simulink model "BMS_SOC"  (R2025b)
settings: Solver=ode4  StartTime=0.0  StopTime=7000  FixedStep=0.1  MaxStep=1  RelTol=1e-3
undefined symbols (not defined in the file or in its folder): batt, cell, metadata
settings Model: SimulationMode=accelerator  Creator=39327  LastModifiedBy=faxio
settings DebuggingCC: UnconnectedInputMsg=warning  UnconnectedOutputMsg=warning  UnconnectedLineMsg=warning
settings ModelReferenceCC: EnableRefExpFcnMdlSchedulingChecks=on
settings RTWCC: GPUComputeCapability=3.5  DLArmComputeVersion=19.05

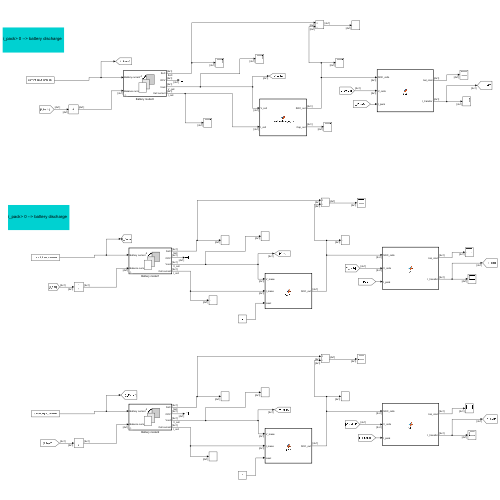
[thumbnail: Simulink's stored preview of the top-level diagram]
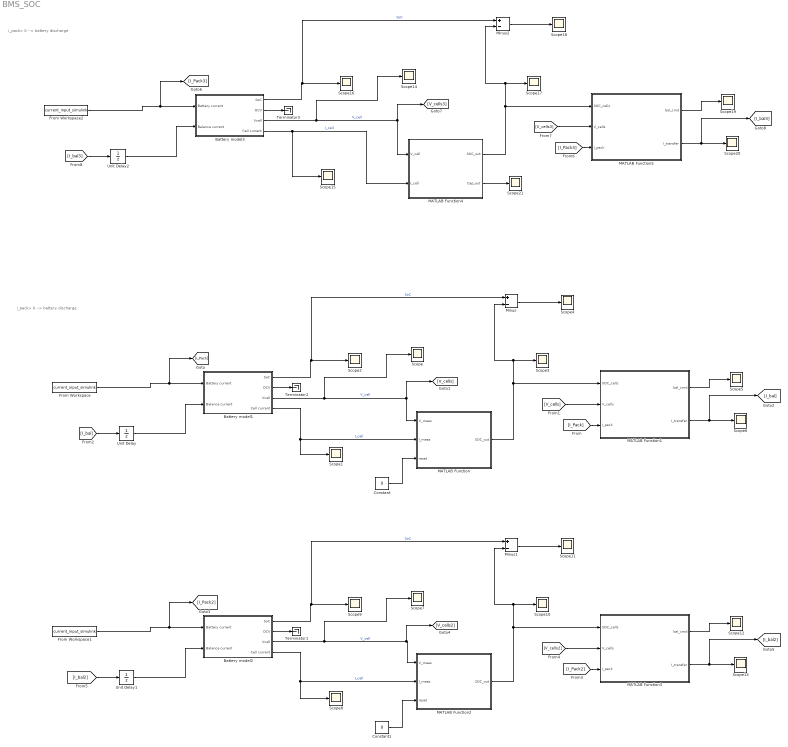
== system BMS_SOC ==
  note: i_pack> 0 --> battery discharge
  note: i_pack> 0 --> battery discharge
  Battery model1 : Subsystem  mask{Soc_init=batt.soc0, Qcell=batt.c_cell, R0_data=batt.r0, R1=batt.r1, C1=batt.c1, ocv_data=cell.ocv, soc_data=cell.soc}
      mask prompts: Soc_init "initial SoC [N_cell*1]"; Qcell "cell capacity [N_cell*1]"; R0_data "R0 [Ncell*soc_pnt]"; R1 "R1[not used here]"; C1 "C1[not used here]"; ocv_data "ocv_data [1*soc_pnt]"; soc_data "soc_data [1*soc_pnt]"
      mask DialogControl DescGroupVar Prompt: Battery model composed of Ncell
      mask DialogControl DescTextVar Prompt: the SoC varies in range 0-1.  Cell number is defined with the dimension of "cell capacity"[N_cell]
  Battery model2 : Subsystem  mask{Soc_init=batt.soc0, Qcell=batt.c_cell, R0_data=batt.r0, R1=batt.r1, C1=batt.c1, ocv_data=cell.ocv, soc_data=cell.soc}
      mask prompts: Soc_init "initial SoC [N_cell*1]"; Qcell "cell capacity [N_cell*1]"; R0_data "R0 [Ncell*soc_pnt]"; R1 "R1[not used here]"; C1 "C1[not used here]"; ocv_data "ocv_data [1*soc_pnt]"; soc_data "soc_data [1*soc_pnt]"
      mask DialogControl DescGroupVar Prompt: Battery model composed of Ncell
      mask DialogControl DescTextVar Prompt: the SoC varies in range 0-1.  Cell number is defined with the dimension of "cell capacity"[N_cell]
  Battery model3 : Subsystem  mask{Soc_init=batt.soc0, Qcell=batt.c_cell, R0_data=batt.r0, R1=batt.r1, C1=batt.c1, ocv_data=cell.ocv, soc_data=cell.soc}
      mask prompts: Soc_init "initial SoC [N_cell*1]"; Qcell "cell capacity [N_cell*1]"; R0_data "R0 [Ncell*soc_pnt]"; R1 "R1[not used here]"; C1 "C1[not used here]"; ocv_data "ocv_data [1*soc_pnt]"; soc_data "soc_data [1*soc_pnt]"
      mask DialogControl DescGroupVar Prompt: Battery model composed of Ncell
      mask DialogControl DescTextVar Prompt: the SoC varies in range 0-1.  Cell number is defined with the dimension of "cell capacity"[N_cell]
  Constant : Constant  Value=0
  Constant1 : Constant  Value=0
  From Workspace : FromWorkspace  VariableName=current_input_simulink  SampleTime=1
  From Workspace1 : FromWorkspace  VariableName=current_input_simulink  SampleTime=1
  From Workspace2 : FromWorkspace  VariableName=current_input_simulink  SampleTime=1
  MATLAB Function : MATLAB Function  TreatAsAtomicUnit=on
  MATLAB Function1 : MATLAB Function  TreatAsAtomicUnit=on  SystemSampleTime=0.1
  MATLAB Function2 : MATLAB Function  TreatAsAtomicUnit=on
  MATLAB Function3 : MATLAB Function  TreatAsAtomicUnit=on  SystemSampleTime=0.1
  MATLAB Function4 : MATLAB Function  TreatAsAtomicUnit=on
  MATLAB Function5 : MATLAB Function  TreatAsAtomicUnit=on  SystemSampleTime=0.1
  Minus : Sum  Inputs=+-
  Minus1 : Sum  Inputs=+-
  Minus2 : Sum  Inputs=+-
  Scope{,1..21} (22 alike) : Scope
      Scope settings: ActiveDisplayYMinimum=3.2688273744129139  ActiveDisplayYMaximum=4.3528683057854645
      Scope1 settings: ActiveDisplayYMinimum=-4.7084210256264356  ActiveDisplayYMaximum=4.9676023361807147
      Scope10 settings: ActiveDisplayYMinimum=-0.1  ActiveDisplayYMaximum=1.1  DataLoggingVariableName=ScopeData7
      Scope11 settings: ActiveDisplayYMinimum=-0.15496450956014618  ActiveDisplayYMaximum=0.21781817172296922  DataLoggingVariableName=ScopeData8
      Scope12 settings: ActiveDisplayYMinimum=-1.2378278494765407  ActiveDisplayYMaximum=1.1192335784275058  DataLoggingVariableName=ScopeData9
      Scope13 settings: ActiveDisplayYMinimum=-1.1600000000000001  ActiveDisplayYMaximum=1.24  DataLoggingVariableName=ScopeData10
      Scope14 settings: ActiveDisplayYMinimum=3.2688273744129139  ActiveDisplayYMaximum=4.3528683057854645  DataLoggingVariableName=ScopeData14
      Scope15 settings: ActiveDisplayYMinimum=-4.7084210256264356  ActiveDisplayYMaximum=4.9676023361807147  DataLoggingVariableName=ScopeData15
      Scope16 settings: ActiveDisplayYMinimum=-0.1  ActiveDisplayYMaximum=1.1  DataLoggingVariableName=ScopeData16
      Scope17 settings: ActiveDisplayYMinimum=0.92795123772963251  ActiveDisplayYMaximum=1.0349099222905718  DataLoggingVariableName=ScopeData17
      Scope18 settings: ActiveDisplayYMinimum=-0.30283794359420108  ActiveDisplayYMaximum=0.25636016397696909  DataLoggingVariableName=ScopeData18
      Scope19 settings: ActiveDisplayYMinimum=-1.2378278494765407  ActiveDisplayYMaximum=1.1192335784275058  DataLoggingVariableName=ScopeData19
      Scope2 settings: ActiveDisplayYMinimum=-0.1  ActiveDisplayYMaximum=1.1  DataLoggingVariableName=ScopeData2
      Scope20 settings: ActiveDisplayYMinimum=-0.32080851306321917  ActiveDisplayYMaximum=0.28672639786307896  DataLoggingVariableName=ScopeData20
      Scope21 settings: ActiveDisplayYMinimum=-2.039376682993602E+9  ActiveDisplayYMaximum=1.6277220397698671E+10  DataLoggingVariableName=ScopeData21
      Scope3 settings: ActiveDisplayYMinimum=-0.1  ActiveDisplayYMaximum=1.1  DataLoggingVariableName=ScopeData3
      Scope4 settings: ActiveDisplayYMinimum=-0.015721734219682579  ActiveDisplayYMaximum=0.063471743751515083  DataLoggingVariableName=ScopeData4
      Scope5 settings: ActiveDisplayYMinimum=-1.2378278494765407  ActiveDisplayYMaximum=1.1192335784275058  DataLoggingVariableName=ScopeData5
      Scope6 settings: ActiveDisplayYMinimum=-0.32080851306321917  ActiveDisplayYMaximum=0.28672639786307896  DataLoggingVariableName=ScopeData6
      Scope7 settings: ActiveDisplayYMinimum=3.2688273744129139  ActiveDisplayYMaximum=4.3528683057854645  DataLoggingVariableName=ScopeData11
      Scope8 settings: ActiveDisplayYMinimum=-4.7084210256264356  ActiveDisplayYMaximum=4.9676023361807147  DataLoggingVariableName=ScopeData12
      Scope9 settings: ActiveDisplayYMinimum=-0.1  ActiveDisplayYMaximum=1.1  DataLoggingVariableName=ScopeData13
  Terminator1 : Terminator
  Terminator2 : Terminator
  Terminator3 : Terminator
  Unit Delay : UnitDelay  SampleTime=-1  HasFrameUpgradeWarning=on
  Unit Delay1 : UnitDelay  SampleTime=-1  HasFrameUpgradeWarning=on
  Unit Delay2 : UnitDelay  SampleTime=-1  HasFrameUpgradeWarning=on
  wires:
  Battery model1/2(OCV) -> Terminator2/1
  From Workspace/1 -> [I_Pack], Battery model1/1(Battery current)
  Battery model1/1(SoC) -> Minus/1, Scope2/1  "SoC"
  [I_bal] -> Unit Delay/1
  Battery model1/3(Vcell) -> Scope/1, [V_cells], MATLAB Function/1(V_meas)  "V_cell"
  Battery model1/4(Cell current) -> Scope1/1, MATLAB Function/2(I_meas)  "I_cell"
  MATLAB Function/1(SOC_out) -> Minus/2, Scope3/1, MATLAB Function1/1(SOC_cells)
  [I_Pack] -> MATLAB Function1/3(I_pack)
  [V_cells] -> MATLAB Function1/2(V_cells)
  MATLAB Function1/2(I_transfer) -> Scope6/1, [I_bal]
  MATLAB Function1/1(bal_cmd) -> Scope5/1
  Unit Delay/1 -> Battery model1/2(Balance current)
  Minus/1 -> Scope4/1
  Minus1/1 -> Scope11/1
  [I_Pack2] -> MATLAB Function3/3(I_pack)
  [V_cells2] -> MATLAB Function3/2(V_cells)
  Battery model2/3(Vcell) -> Scope7/1, MATLAB Function2/1(V_meas), [V_cells2]  "V_cell"
  Battery model2/4(Cell current) -> MATLAB Function2/2(I_meas), Scope8/1  "I_cell"
  From Workspace1/1 -> [I_Pack2], Battery model2/1(Battery current)
  [I_bal2] -> Unit Delay1/1
  MATLAB Function3/1(bal_cmd) -> Scope12/1
  Unit Delay1/1 -> Battery model2/2(Balance current)
  MATLAB Function2/1(SOC_out) -> Minus1/2, Scope10/1, MATLAB Function3/1(SOC_cells)
  Battery model2/2(OCV) -> Terminator1/1
  Battery model2/1(SoC) -> Minus1/1, Scope9/1  "SoC"
  Constant1/1 -> MATLAB Function2/3(reset)
  MATLAB Function3/2(I_transfer) -> Scope13/1, [I_bal2]
  MATLAB Function5/2(I_transfer) -> Scope20/1, [I_bal3]
  Battery model3/3(Vcell) -> Scope14/1, [V_cells3], MATLAB Function4/1(V_cell)  "V_cell"
  [I_bal3] -> Unit Delay2/1
  Unit Delay2/1 -> Battery model3/2(Balance current)
  From Workspace2/1 -> [I_Pack3], Battery model3/1(Battery current)
  Battery model3/4(Cell current) -> MATLAB Function4/2(I_cell), Scope15/1  "I_cell"
  [V_cells3] -> MATLAB Function5/2(V_cells)
  [I_Pack3] -> MATLAB Function5/3(I_pack)
  MATLAB Function5/1(bal_cmd) -> Scope19/1
  MATLAB Function4/1(SOC_out) -> Minus2/2, Scope17/1, MATLAB Function5/1(SOC_cells)
  Battery model3/1(SoC) -> Minus2/1, Scope16/1  "SoC"
  Minus2/1 -> Scope18/1
  Battery model3/2(OCV) -> Terminator3/1
  Constant/1 -> MATLAB Function/3(reset)
  MATLAB Function4/2(Cap_out) -> Scope21/1

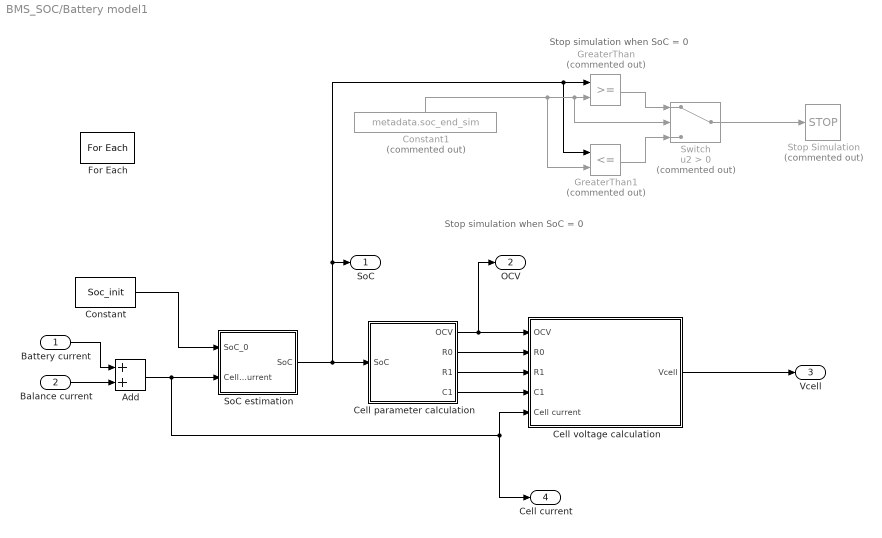
== system BMS_SOC/Battery model1 ==
  note: Stop simulation when SoC = 0
  note: Stop simulation when SoC = 0
  Battery current : Inport
  Balance current : Inport  Port=2  Partition=on  PartitionDimension=1  PartitionWidth=1  PartitionOffset=0
  Add : Sum
  Cell parameter calculation : Subsystem
  Cell voltage calculation : Subsystem
  Constant : Constant  Value=Soc_init
  Constant1 : Constant  Commented=on  Value=metadata.soc_end_sim
  For Each : ForEach  DisableCoverage=on  IterateSubsysMaskParameter=on,on,on,off,off,off,off
  GreaterThan : RelationalOperator  Commented=on  OutDataTypeStr=boolean  RndMeth=Simplest  InputSameDT=off
  GreaterThan1 : RelationalOperator  Commented=on  Operator=<=  OutDataTypeStr=boolean  RndMeth=Simplest  InputSameDT=off
  SoC estimation : Subsystem
  Stop Simulation : Stop  Commented=on
  Switch : Switch  Commented=on  Criteria=u2 > Threshold  SaturateOnIntegerOverflow=off  InputSameDT=off
  SoC : Outport  ConcatenationDimension=1
  OCV : Outport  Port=2  ConcatenationDimension=1
  Vcell : Outport  Port=3  ConcatenationDimension=1
  Cell current : Outport  Port=4  ConcatenationDimension=1
  wires:
  Add/1 -> Cell voltage calculation/5(Cell current), Cell current/1, SoC estimation/2(Cell current)
  Constant/1 -> SoC estimation/1(SoC_0)
  SoC estimation/1(SoC) -> GreaterThan/1, GreaterThan1/1, SoC/1, Cell parameter calculation/1(SoC)
  Cell parameter calculation/4(C1) -> Cell voltage calculation/4(C1)
  Cell parameter calculation/3(R1) -> Cell voltage calculation/3(R1)
  Cell parameter calculation/2(R0) -> Cell voltage calculation/2(R0)
  Cell parameter calculation/1(OCV) -> OCV/1, Cell voltage calculation/1(OCV)
  Cell voltage calculation/1(Vcell) -> Vcell/1
  Battery current/1 -> Add/1
  Balance current/1 -> Add/2
  Constant1/1 -> GreaterThan/2, Switch/2, GreaterThan1/2
  Switch/1 -> Stop Simulation/1
  GreaterThan/1 -> Switch/1
  GreaterThan1/1 -> Switch/3

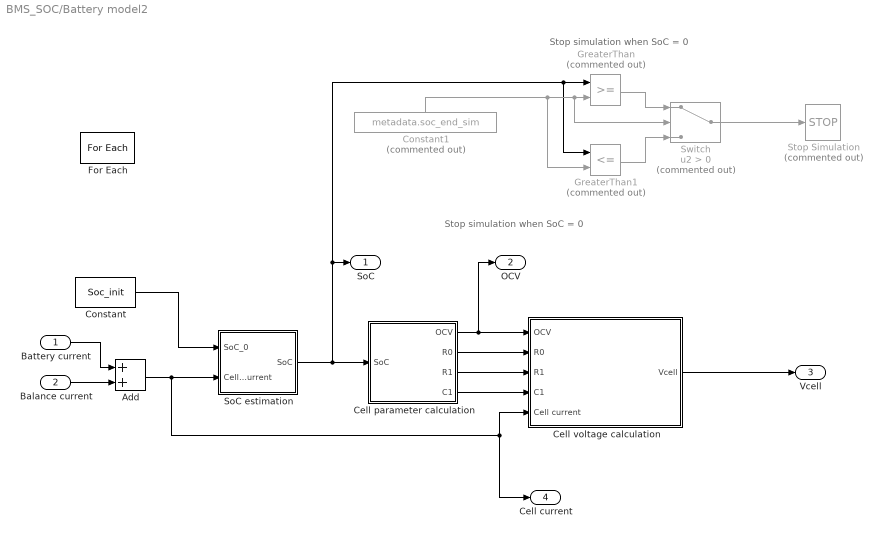
== system BMS_SOC/Battery model2 ==
  note: Stop simulation when SoC = 0
  note: Stop simulation when SoC = 0
  Battery current : Inport
  Balance current : Inport  Port=2  Partition=on  PartitionDimension=1  PartitionWidth=1  PartitionOffset=0
  Add : Sum
  Cell parameter calculation : Subsystem
  Cell voltage calculation : Subsystem
  Constant : Constant  Value=Soc_init
  Constant1 : Constant  Commented=on  Value=metadata.soc_end_sim
  For Each : ForEach  DisableCoverage=on  IterateSubsysMaskParameter=on,on,on,off,off,off,off
  GreaterThan : RelationalOperator  Commented=on  OutDataTypeStr=boolean  RndMeth=Simplest  InputSameDT=off
  GreaterThan1 : RelationalOperator  Commented=on  Operator=<=  OutDataTypeStr=boolean  RndMeth=Simplest  InputSameDT=off
  SoC estimation : Subsystem
  Stop Simulation : Stop  Commented=on
  Switch : Switch  Commented=on  Criteria=u2 > Threshold  SaturateOnIntegerOverflow=off  InputSameDT=off
  SoC : Outport  ConcatenationDimension=1
  OCV : Outport  Port=2  ConcatenationDimension=1
  Vcell : Outport  Port=3  ConcatenationDimension=1
  Cell current : Outport  Port=4  ConcatenationDimension=1
  wires:
  Add/1 -> Cell voltage calculation/5(Cell current), Cell current/1, SoC estimation/2(Cell current)
  Constant/1 -> SoC estimation/1(SoC_0)
  SoC estimation/1(SoC) -> GreaterThan/1, GreaterThan1/1, SoC/1, Cell parameter calculation/1(SoC)
  Cell parameter calculation/4(C1) -> Cell voltage calculation/4(C1)
  Cell parameter calculation/3(R1) -> Cell voltage calculation/3(R1)
  Cell parameter calculation/2(R0) -> Cell voltage calculation/2(R0)
  Cell parameter calculation/1(OCV) -> OCV/1, Cell voltage calculation/1(OCV)
  Cell voltage calculation/1(Vcell) -> Vcell/1
  Battery current/1 -> Add/1
  Balance current/1 -> Add/2
  Constant1/1 -> GreaterThan/2, Switch/2, GreaterThan1/2
  Switch/1 -> Stop Simulation/1
  GreaterThan/1 -> Switch/1
  GreaterThan1/1 -> Switch/3

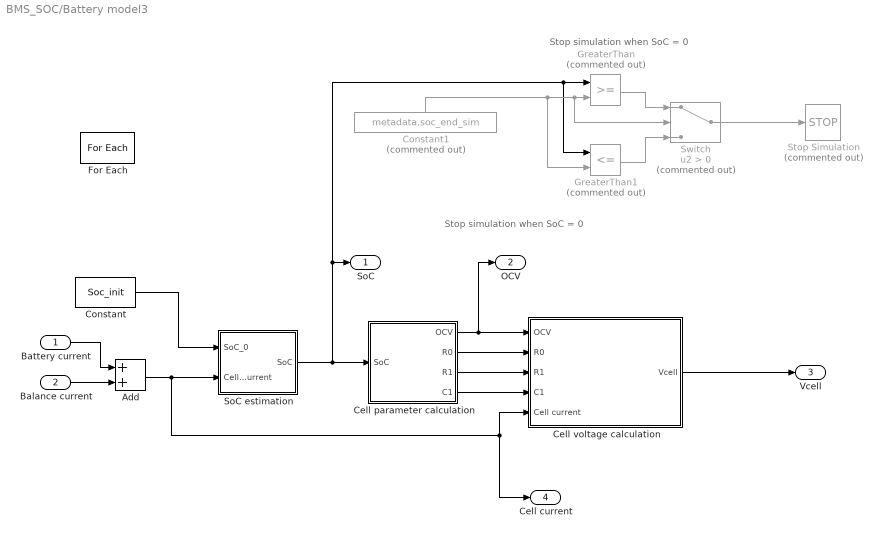
== system BMS_SOC/Battery model3 ==
  note: Stop simulation when SoC = 0
  note: Stop simulation when SoC = 0
  Battery current : Inport
  Balance current : Inport  Port=2  Partition=on  PartitionDimension=1  PartitionWidth=1  PartitionOffset=0
  Add : Sum
  Cell parameter calculation : Subsystem
  Cell voltage calculation : Subsystem
  Constant : Constant  Value=Soc_init
  Constant1 : Constant  Commented=on  Value=metadata.soc_end_sim
  For Each : ForEach  DisableCoverage=on  IterateSubsysMaskParameter=on,on,on,off,off,off,off
  GreaterThan : RelationalOperator  Commented=on  OutDataTypeStr=boolean  RndMeth=Simplest  InputSameDT=off
  GreaterThan1 : RelationalOperator  Commented=on  Operator=<=  OutDataTypeStr=boolean  RndMeth=Simplest  InputSameDT=off
  SoC estimation : Subsystem
  Stop Simulation : Stop  Commented=on
  Switch : Switch  Commented=on  Criteria=u2 > Threshold  SaturateOnIntegerOverflow=off  InputSameDT=off
  SoC : Outport  ConcatenationDimension=1
  OCV : Outport  Port=2  ConcatenationDimension=1
  Vcell : Outport  Port=3  ConcatenationDimension=1
  Cell current : Outport  Port=4  ConcatenationDimension=1
  wires:
  Add/1 -> Cell voltage calculation/5(Cell current), Cell current/1, SoC estimation/2(Cell current)
  Constant/1 -> SoC estimation/1(SoC_0)
  SoC estimation/1(SoC) -> GreaterThan/1, GreaterThan1/1, SoC/1, Cell parameter calculation/1(SoC)
  Cell parameter calculation/4(C1) -> Cell voltage calculation/4(C1)
  Cell parameter calculation/3(R1) -> Cell voltage calculation/3(R1)
  Cell parameter calculation/2(R0) -> Cell voltage calculation/2(R0)
  Cell parameter calculation/1(OCV) -> OCV/1, Cell voltage calculation/1(OCV)
  Cell voltage calculation/1(Vcell) -> Vcell/1
  Battery current/1 -> Add/1
  Balance current/1 -> Add/2
  Constant1/1 -> GreaterThan/2, Switch/2, GreaterThan1/2
  Switch/1 -> Stop Simulation/1
  GreaterThan/1 -> Switch/1
  GreaterThan1/1 -> Switch/3

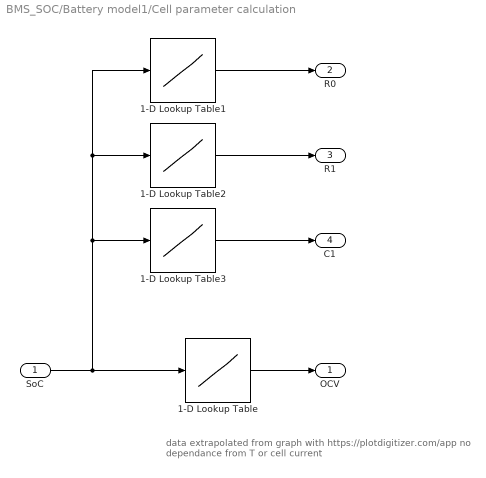
== system BMS_SOC/Battery model1/Cell parameter calculation ==
  note: data extrapolated from graph with https://plotdigitizer.com/app
      |
      | no dependance from T or cell current
  SoC : Inport
  1-D Lookup Table : Lookup_n-D  NumberOfTableDimensions=1  BreakpointsForDimension1=cell.soc  Table=cell.ocv  InternalRulePriority=Speed  RndMeth=Simplest
  1-D Lookup Table1 : Lookup_n-D  NumberOfTableDimensions=1  BreakpointsForDimension1=cell.soc  Table=cell.r0  InternalRulePriority=Speed  RndMeth=Simplest
  1-D Lookup Table2 : Lookup_n-D  NumberOfTableDimensions=1  BreakpointsForDimension1=cell.soc  Table=cell.r1  InternalRulePriority=Speed  RndMeth=Simplest
  1-D Lookup Table3 : Lookup_n-D  NumberOfTableDimensions=1  BreakpointsForDimension1=cell.soc  Table=cell.c1  InternalRulePriority=Speed  RndMeth=Simplest
  OCV : Outport
  R0 : Outport  Port=2
  R1 : Outport  Port=3
  C1 : Outport  Port=4
  wires:
  1-D Lookup Table/1 -> OCV/1
  SoC/1 -> 1-D Lookup Table3/1, 1-D Lookup Table2/1, 1-D Lookup Table1/1, 1-D Lookup Table/1
  1-D Lookup Table1/1 -> R0/1
  1-D Lookup Table3/1 -> C1/1
  1-D Lookup Table2/1 -> R1/1

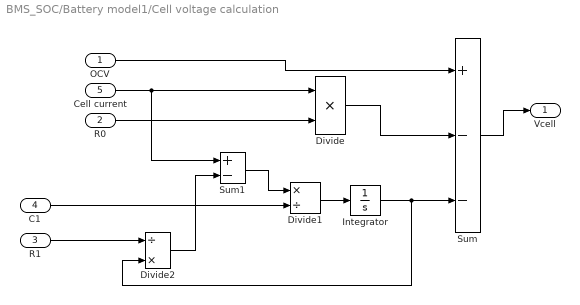
== system BMS_SOC/Battery model1/Cell voltage calculation ==
  OCV : Inport
  R0 : Inport  Port=2
  R1 : Inport  Port=3
  C1 : Inport  Port=4
  Cell current : Inport  Port=5
  Divide : Product  Inputs=**
  Divide1 : Product  Inputs=*/
  Divide2 : Product  Inputs=/*
  Integrator : Integrator
  Sum : Sum  Inputs=+--
  Sum1 : Sum  Inputs=+-
  Vcell : Outport
  wires:
  Sum/1 -> Vcell/1
  OCV/1 -> Sum/1
  Divide/1 -> Sum/2
  Cell current/1 -> Sum1/1, Divide/1
  R0/1 -> Divide/2
  Divide1/1 -> Integrator/1
  Integrator/1 -> Sum/3, Divide2/2
  Sum1/1 -> Divide1/1
  Divide2/1 -> Sum1/2
  C1/1 -> Divide1/2
  R1/1 -> Divide2/1

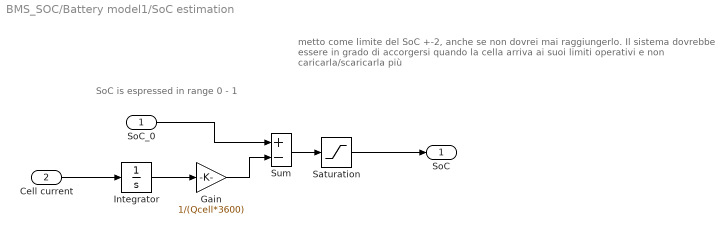
== system BMS_SOC/Battery model1/SoC estimation ==
  note: metto come limite del SoC +-2, anche se non dovrei mai raggiungerlo. Il sistema dovrebbe essere in grado di accorgersi quando la cella arriva ai suoi limiti operativi e non caricarla/scaricarla più
  note: SoC is espressed in range 0 - 1
  SoC_0 : Inport
  Cell current : Inport  Port=2
  Gain : Gain  Gain=1/(Qcell*3600)
  Integrator : Integrator
  Saturation : Saturate  UpperLimit=2  LowerLimit=-2
  Sum : Sum  Inputs=+-
  SoC : Outport
  wires:
  Saturation/1 -> SoC/1
  Integrator/1 -> Gain/1
  Cell current/1 -> Integrator/1
  Sum/1 -> Saturation/1
  Gain/1 -> Sum/2
  SoC_0/1 -> Sum/1

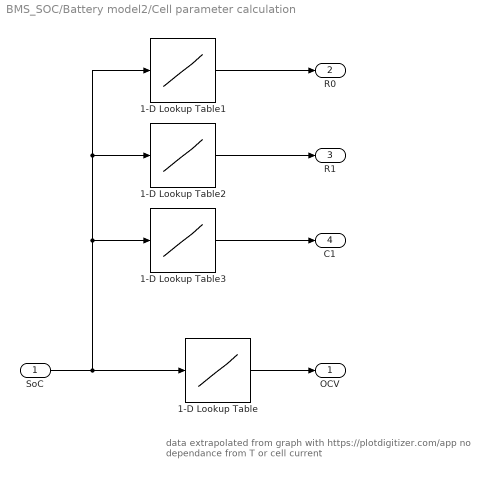
== system BMS_SOC/Battery model2/Cell parameter calculation ==
  note: data extrapolated from graph with https://plotdigitizer.com/app
      |
      | no dependance from T or cell current
  SoC : Inport
  1-D Lookup Table : Lookup_n-D  NumberOfTableDimensions=1  BreakpointsForDimension1=cell.soc  Table=cell.ocv  InternalRulePriority=Speed  RndMeth=Simplest
  1-D Lookup Table1 : Lookup_n-D  NumberOfTableDimensions=1  BreakpointsForDimension1=cell.soc  Table=cell.r0  InternalRulePriority=Speed  RndMeth=Simplest
  1-D Lookup Table2 : Lookup_n-D  NumberOfTableDimensions=1  BreakpointsForDimension1=cell.soc  Table=cell.r1  InternalRulePriority=Speed  RndMeth=Simplest
  1-D Lookup Table3 : Lookup_n-D  NumberOfTableDimensions=1  BreakpointsForDimension1=cell.soc  Table=cell.c1  InternalRulePriority=Speed  RndMeth=Simplest
  OCV : Outport
  R0 : Outport  Port=2
  R1 : Outport  Port=3
  C1 : Outport  Port=4
  wires:
  1-D Lookup Table/1 -> OCV/1
  SoC/1 -> 1-D Lookup Table3/1, 1-D Lookup Table2/1, 1-D Lookup Table1/1, 1-D Lookup Table/1
  1-D Lookup Table1/1 -> R0/1
  1-D Lookup Table3/1 -> C1/1
  1-D Lookup Table2/1 -> R1/1

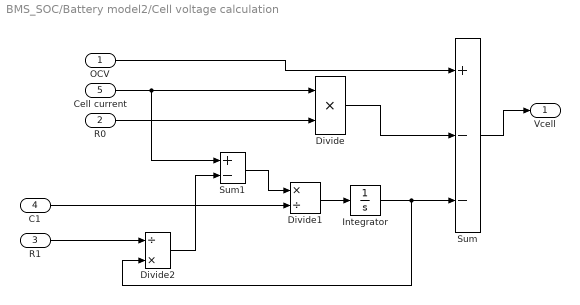
== system BMS_SOC/Battery model2/Cell voltage calculation ==
  OCV : Inport
  R0 : Inport  Port=2
  R1 : Inport  Port=3
  C1 : Inport  Port=4
  Cell current : Inport  Port=5
  Divide : Product  Inputs=**
  Divide1 : Product  Inputs=*/
  Divide2 : Product  Inputs=/*
  Integrator : Integrator
  Sum : Sum  Inputs=+--
  Sum1 : Sum  Inputs=+-
  Vcell : Outport
  wires:
  Sum/1 -> Vcell/1
  OCV/1 -> Sum/1
  Divide/1 -> Sum/2
  Cell current/1 -> Sum1/1, Divide/1
  R0/1 -> Divide/2
  Divide1/1 -> Integrator/1
  Integrator/1 -> Sum/3, Divide2/2
  Sum1/1 -> Divide1/1
  Divide2/1 -> Sum1/2
  C1/1 -> Divide1/2
  R1/1 -> Divide2/1

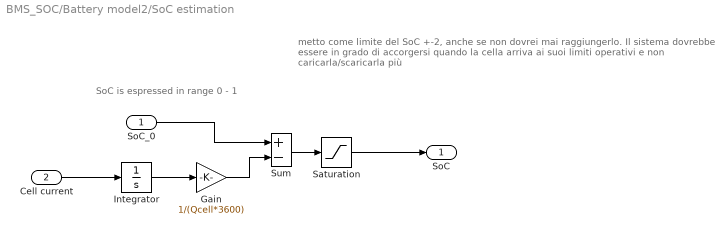
== system BMS_SOC/Battery model2/SoC estimation ==
  note: metto come limite del SoC +-2, anche se non dovrei mai raggiungerlo. Il sistema dovrebbe essere in grado di accorgersi quando la cella arriva ai suoi limiti operativi e non caricarla/scaricarla più
  note: SoC is espressed in range 0 - 1
  SoC_0 : Inport
  Cell current : Inport  Port=2
  Gain : Gain  Gain=1/(Qcell*3600)
  Integrator : Integrator
  Saturation : Saturate  UpperLimit=2  LowerLimit=-2
  Sum : Sum  Inputs=+-
  SoC : Outport
  wires:
  Saturation/1 -> SoC/1
  Integrator/1 -> Gain/1
  Cell current/1 -> Integrator/1
  Sum/1 -> Saturation/1
  Gain/1 -> Sum/2
  SoC_0/1 -> Sum/1

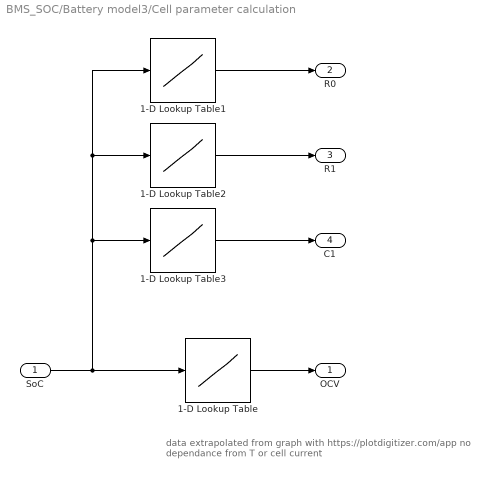
== system BMS_SOC/Battery model3/Cell parameter calculation ==
  note: data extrapolated from graph with https://plotdigitizer.com/app
      |
      | no dependance from T or cell current
  SoC : Inport
  1-D Lookup Table : Lookup_n-D  NumberOfTableDimensions=1  BreakpointsForDimension1=cell.soc  Table=cell.ocv  InternalRulePriority=Speed  RndMeth=Simplest
  1-D Lookup Table1 : Lookup_n-D  NumberOfTableDimensions=1  BreakpointsForDimension1=cell.soc  Table=cell.r0  InternalRulePriority=Speed  RndMeth=Simplest
  1-D Lookup Table2 : Lookup_n-D  NumberOfTableDimensions=1  BreakpointsForDimension1=cell.soc  Table=cell.r1  InternalRulePriority=Speed  RndMeth=Simplest
  1-D Lookup Table3 : Lookup_n-D  NumberOfTableDimensions=1  BreakpointsForDimension1=cell.soc  Table=cell.c1  InternalRulePriority=Speed  RndMeth=Simplest
  OCV : Outport
  R0 : Outport  Port=2
  R1 : Outport  Port=3
  C1 : Outport  Port=4
  wires:
  1-D Lookup Table/1 -> OCV/1
  SoC/1 -> 1-D Lookup Table3/1, 1-D Lookup Table2/1, 1-D Lookup Table1/1, 1-D Lookup Table/1
  1-D Lookup Table1/1 -> R0/1
  1-D Lookup Table3/1 -> C1/1
  1-D Lookup Table2/1 -> R1/1

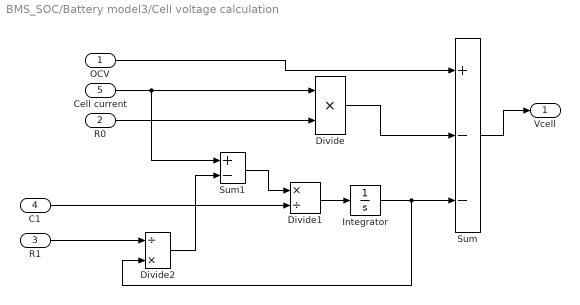
== system BMS_SOC/Battery model3/Cell voltage calculation ==
  OCV : Inport
  R0 : Inport  Port=2
  R1 : Inport  Port=3
  C1 : Inport  Port=4
  Cell current : Inport  Port=5
  Divide : Product  Inputs=**
  Divide1 : Product  Inputs=*/
  Divide2 : Product  Inputs=/*
  Integrator : Integrator
  Sum : Sum  Inputs=+--
  Sum1 : Sum  Inputs=+-
  Vcell : Outport
  wires:
  Sum/1 -> Vcell/1
  OCV/1 -> Sum/1
  Divide/1 -> Sum/2
  Cell current/1 -> Sum1/1, Divide/1
  R0/1 -> Divide/2
  Divide1/1 -> Integrator/1
  Integrator/1 -> Sum/3, Divide2/2
  Sum1/1 -> Divide1/1
  Divide2/1 -> Sum1/2
  C1/1 -> Divide1/2
  R1/1 -> Divide2/1

== system BMS_SOC/Battery model3/SoC estimation ==
  note: metto come limite del SoC +-2, anche se non dovrei mai raggiungerlo. Il sistema dovrebbe essere in grado di accorgersi quando la cella arriva ai suoi limiti operativi e non caricarla/scaricarla più
  note: SoC is espressed in range 0 - 1
  SoC_0 : Inport
  Cell current : Inport  Port=2
  Gain : Gain  Gain=1/(Qcell*3600)
  Integrator : Integrator
  Saturation : Saturate  UpperLimit=2  LowerLimit=-2
  Sum : Sum  Inputs=+-
  SoC : Outport
  wires:
  Saturation/1 -> SoC/1
  Integrator/1 -> Gain/1
  Cell current/1 -> Integrator/1
  Sum/1 -> Saturation/1
  Gain/1 -> Sum/2
  SoC_0/1 -> Sum/1

== matlab function BMS_SOC/MATLAB Function1 ==
  settings: updateMethod=DISCRETE  sampleTime=0.1
  data: SOC_cells input; bal_cmd output; V_cells input; I_pack input; I_transfer output; batt_param parameter
function [bal_cmd, I_transfer] = BAL(SOC_cells, V_cells, I_pack, batt_param)

    n_cells = 4;
    
    I_bal_max = batt_param.I_bal_max;
    eta_dcdc = batt_param.eta_dcdc;
    SOC_threshold = batt_param.SOC_threshold;
    V_min_bal = batt_param.V_min_bal;
    V_max_bal = batt_param.V_max_bal;
    
    bal_cmd = zeros(4, 1);
    I_transfer = zeros(4, 1);
    
    % Trova SOC max e min
    SOC_min = SOC_cells(1);
    SOC_max = SOC_cells(1);
    idx_min = 1;
    idx_max = 1;
    
    for k = 1:n_cells
        if SOC_cells(k) < SOC_min
            SOC_min = SOC_cells(k);
            idx_min = k;
        end
        if SOC_cells(k) > SOC_max
            SOC_max = SOC_cells(k);
            idx_max = k;
        end
    end
    
    SOC_range = SOC_max - SOC_min;
    
    % Bilancia se necessario
    if SOC_range > SOC_threshold
        
        V_source = V_cells(idx_max);
        V_dest = V_cells(idx_min);
        
        safe = (V_source > V_min_bal) && (V_source < V_max_bal) && ... 
               (V_dest > V_min_bal) && (V_dest < V_max_bal);
        
        if safe
            I_bal = min(5 * SOC_range * I_bal_max, I_bal_max);
            
            bal_cmd(idx_max) = 1;
            I_transfer(idx_max) = I_bal;
            
            bal_cmd(idx_min) = -1;
            I_transfer(idx_min) = -I_bal * eta_dcdc;
        end
    end
    
end

== matlab function BMS_SOC/MATLAB Function ==
  settings: updateMethod=DISCRETE  sampleTime=0.1
  data: V_meas input; SOC_out output size=[4 1]; I_meas input; reset input; batt_param parameter
function SOC_out  = AEKF(V_meas, I_meas, reset,batt_param)

% Ingressi:
%   V_meas - Vettore tensioni misurate [n_cells x 1]
%   I_meas - Vettore correnti misurate [n_cells x 1]  
%   reset  - Segnale di reset (boolean)
%
% Uscita:
%   SOC_out - SOC stimato [n_cells x 1]
    
    M=10; %finestra di misura per AEKF
    % Numero di celle 
    n_cells = 4;

    % Parametri batteria
    Ts = 0.1;           % Tempo campionamento [s]
    Q_cell = batt_param.c_cell;        % Capacità [Ah]
    R0_matrix = batt_param.r0;         % Resistenza ohmica [Ohm]
    R1_matrix = batt_param.r1;         % Resistenza RC [Ohm]
    C1_matrix = batt_param.c1;          % Capacità RC [F]
    
    SOC_grid =batt_param.soc(:);
    OCV_tab  =batt_param.ocv(:);

    % Pre-calcola derivata OCV
    n_points = length(SOC_grid);
    dSOC = SOC_grid(2) - SOC_grid(1);
    dOCV_temp = diff(OCV_tab) / dSOC;
    dOCV_tab = zeros(n_points, 1);
    dOCV_tab(1) = dOCV_temp(1);
    for i = 2:n_points-1
        dOCV_tab(i) = dOCV_temp(i);
    end
    dOCV_tab(n_points) = dOCV_temp(n_points-1);
     
    % % Rumore EKF
    % Q_cov = diag([1e-5, 1e-3]);
    % R_var = 0.00001;
    
   persistent SOC_state V1_state P_state H_k_vector Q_cov R_var initialized

if isempty(initialized) || reset
    SOC_state = 0.5 * ones(n_cells,1);
    V1_state  = zeros(n_cells,1);
    P_state   = zeros(2,2,n_cells);
    
    H_k_vector=    zeros(1,M);
    Q_cov = diag([1e-5, 1e-3]);
    R_var = 0.00001;
    
    for k = 1:n_cells
        P_state(:,:,k) = diag([0.05, 0.01]);
    end
    initialized = true;
end

%% PRE-ALLOCAZIONE

SOC_out = zeros(n_cells,1);
    H_k=0;
%% EKF PER OGNI CELLA

for k = 1:n_cells

    % Stato corrente
    x = [SOC_state(k); V1_state(k)];
    P = P_state(:,:,k);

    I_k = I_meas(k);
    V_k = V_meas(k);

    %% PREDIZIONE 
    % Coulomb counting
    SOC_pred = x(1) - (Ts * I_k) / (Q_cell(k) * 3600);
    SOC_pred = max(0, min(1, SOC_pred)); %limito il soc tra 0 e 1

    % ESTRAGGO LA RIGA k DALLA MATRICE E FACCIO L'INTERPOLAZIONE
    R0_row = R0_matrix(k, :);  % Riga k, vettore [1 x 21]
    R1_row = R1_matrix(k, :);  % Riga k, vettore [1 x 21]
    C1_row = C1_matrix(k, :);  % Riga k, vettore [1 x 21]
        
    % Converte a colonna per interp1
    R0_col = R0_row(:);  % [21 x 1]
    R1_col = R1_row(:);  % [21 x 1]
    C1_col = C1_row(:);  % [21 x 1]

    % Interpolazione
    R0 = interp1(SOC_grid, R0_col, SOC_pred, 'linear', 'extrap');
    R1 = interp1(SOC_grid, R1_col, SOC_pred, 'linear', 'extrap');
    C1 = interp1(SOC_grid, C1_col, SOC_pred, 'linear', 'extrap');

    tau1  = R1 * C1;
    alpha = exp(-Ts / tau1);

    % Dinamica RC
    V1_pred = alpha * x(2) + R1 * (1 - alpha) * I_k;

    x_pred = [SOC_pred; V1_pred];

    % Jacobiano stato
    A = [1, 0;
         0, alpha];

    P_pred = A * P * A' + Q_cov;

    %% AGGIORNAMENTO
    OCV  = interp1(SOC_grid, OCV_tab, SOC_pred,"linear","extrap");
    dOCV = interp1(SOC_grid, dOCV_tab, SOC_pred,"linear","extrap");
        
    V_pred = OCV - x_pred(2) - R0 * I_k;
    y_tilde = V_k - V_pred;

    C_mat = [dOCV, -1];

    S = C_mat * P_pred * C_mat' + R_var;
    K = (P_pred * C_mat') / S;

    % Aggiornamento stato
    x_upd = x_pred + K * y_tilde;
    x_upd(1) = max(0, min(1, x_upd(1)));

    % Aggiornamento covarianza
    I2 = eye(2);
    P_upd = (I2 - K * C_mat) * P_pred;

    H_k_vector=circshift(H_k_vector,1);
    H_k_vector(1)=y_tilde*y_tilde';
    if H_k_vector(M)~=0
        H_k=sum(H_k_vector)/M;
        Q_cov=K*H_k*K';
        R_var=H_k-C_mat*P_upd*C_mat';
    end
    %% SALVATAGGIO 
    SOC_state(k) = x_upd(1);
    V1_state(k)  = x_upd(2);
    P_state(:,:,k) = P_upd;



    SOC_out(k) = x_upd(1);
        
end
end

== matlab function BMS_SOC/MATLAB Function2 ==
  settings: updateMethod=DISCRETE  sampleTime=0.1
  data: V_meas input; SOC_out output size=[4 1]; I_meas input; reset input; batt_param parameter
function SOC_out  = EKF(V_meas, I_meas, reset,batt_param)

% Ingressi:
%   V_meas - Vettore tensioni misurate [n_cells x 1]
%   I_meas - Vettore correnti misurate [n_cells x 1]  
%   reset  - Segnale di reset (boolean)
%
% Uscita:
%   SOC_out - SOC stimato [n_cells x 1]

    % Numero di celle 
    n_cells = 4;

    % Parametri batteria (CALIBRARE PER LE VOSTRE CELLE)
    Ts = 0.1;           % Tempo campionamento [s]
    Q_cell = batt_param.c_cell;        % Capacità [Ah]
    R0_matrix = batt_param.r0;         % Resistenza ohmica [Ohm]
    R1_matrix = batt_param.r1;         % Resistenza RC [Ohm]
    C1_matrix = batt_param.c1;          % Capacità RC [F]
    
    SOC_grid =batt_param.soc(:);
    OCV_tab  =batt_param.ocv(:);

    % Pre-calcola derivata OCV
    n_points = length(SOC_grid);
    dSOC = SOC_grid(2) - SOC_grid(1);
    dOCV_temp = diff(OCV_tab) / dSOC;
    dOCV_tab = zeros(n_points, 1);
    dOCV_tab(1) = dOCV_temp(1);
    for i = 2:n_points-1
        dOCV_tab(i) = dOCV_temp(i);
    end
    dOCV_tab(n_points) = dOCV_temp(n_points-1);

    % Rumore EKF
    Q_cov = diag([1e-5, 1e-3]);
    R_var = 0.00001;
    
   persistent SOC_state V1_state P_state initialized

if isempty(initialized) || reset
    SOC_state = 0.5 * ones(n_cells,1);
    V1_state  = zeros(n_cells,1);
    P_state   = zeros(2,2,n_cells);
    for k = 1:n_cells
        P_state(:,:,k) = diag([0.05, 0.01]);
    end
    initialized = true;
end

%% PRE-ALLOCAZIONE

SOC_out = zeros(n_cells,1);
%% EKF PER OGNI CELLA

for k = 1:n_cells

    % Stato corrente
    x = [SOC_state(k); V1_state(k)];
    P = P_state(:,:,k);

    I_k = I_meas(k);
    V_k = V_meas(k);

    %% PREDIZIONE 
    % Coulomb counting
    SOC_pred = x(1) - (Ts * I_k) / (Q_cell(k) * 3600);
    SOC_pred = max(0, min(1, SOC_pred));

    % ESTRAI LA RIGA k DALLA MATRICE E INTERPOLA
    R0_row = R0_matrix(k, :);  % Riga k, vettore [1 x 21]
    R1_row = R1_matrix(k, :);  % Riga k, vettore [1 x 21]
    C1_row = C1_matrix(k, :);  % Riga k, vettore [1 x 21]
        
    % Converte a colonna per interp1
    R0_col = R0_row(:);  % [21 x 1]
    R1_col = R1_row(:);  % [21 x 1]
    C1_col = C1_row(:);  % [21 x 1]

    % Interpolazione
    R0 = interp1(SOC_grid, R0_col, SOC_pred, 'linear', 'extrap');
    R1 = interp1(SOC_grid, R1_col, SOC_pred, 'linear', 'extrap');
    C1 = interp1(SOC_grid, C1_col, SOC_pred, 'linear', 'extrap');

    tau1  = R1 * C1;
    alpha = exp(-Ts / tau1);

    % Dinamica RC
    V1_pred = alpha * x(2) + R1 * (1 - alpha) * I_k;

    x_pred = [SOC_pred; V1_pred];

    % Jacobiano stato
    A = [1, 0;
         0, alpha];

    P_pred = A * P * A' + Q_cov;

    %% AGGIORNAMENTO
    OCV  = interp1(SOC_grid, OCV_tab, SOC_pred,"linear","extrap");
    dOCV = interp1(SOC_grid, dOCV_tab, SOC_pred,"linear","extrap");
        
    V_pred = OCV - x_pred(2) - R0 * I_k;
    y_tilde = V_k - V_pred;

    C_mat = [dOCV, -1];

    S = C_mat * P_pred * C_mat' + R_var;
    K = (P_pred * C_mat') / S;

    % Aggiornamento stato
    x_upd = x_pred + K * y_tilde;
    x_upd(1) = max(0, min(1, x_upd(1)));

    % Aggiornamento covarianza
    I2 = eye(2);
    P_upd = (I2 - K * C_mat) * P_pred;

    %% SALVATAGGIO 
    SOC_state(k) = x_upd(1);
    V1_state(k)  = x_upd(2);
    P_state(:,:,k) = P_upd;

    SOC_out(k) = x_upd(1);

end
end

== matlab function BMS_SOC/MATLAB Function3 ==
  settings: updateMethod=DISCRETE  sampleTime=0.1
  data: SOC_cells input; bal_cmd output; V_cells input; I_pack input; I_transfer output; batt_param parameter
function [bal_cmd, I_transfer] = BAL(SOC_cells, V_cells, I_pack, batt_param)

    n_cells = 4;
    
    I_bal_max = batt_param.I_bal_max;
    eta_dcdc = batt_param.eta_dcdc;
    SOC_threshold = batt_param.SOC_threshold;
    V_min_bal = batt_param.V_min_bal;
    V_max_bal = batt_param.V_max_bal;
    
    bal_cmd = zeros(4, 1);
    I_transfer = zeros(4, 1);
    
    % Trova SOC max e min
    SOC_min = SOC_cells(1);
    SOC_max = SOC_cells(1);
    idx_min = 1;
    idx_max = 1;
    
    for k = 1:n_cells
        if SOC_cells(k) < SOC_min
            SOC_min = SOC_cells(k);
            idx_min = k;
        end
        if SOC_cells(k) > SOC_max
            SOC_max = SOC_cells(k);
            idx_max = k;
        end
    end
    
    SOC_range = SOC_max - SOC_min;
    
    % Bilancia se necessario
    if SOC_range > SOC_threshold
        
        V_source = V_cells(idx_max);
        V_dest = V_cells(idx_min);
        
        safe = (V_source > V_min_bal) && (V_source < V_max_bal) && ... 
               (V_dest > V_min_bal) && (V_dest < V_max_bal);
        
        if safe
            I_bal = min(5 * SOC_range * I_bal_max, I_bal_max);
            
            bal_cmd(idx_max) = 1;
            I_transfer(idx_max) = I_bal;
            
            bal_cmd(idx_min) = -1;
            I_transfer(idx_min) = -I_bal * eta_dcdc;
        end
    end
    
end

== matlab function BMS_SOC/MATLAB Function4 ==
  settings: updateMethod=DISCRETE  sampleTime=0.1
  data: SOC_out output size=[4 1]; Cap_out output; V_cell input; I_cell input; batt_param parameter
function [SOC_out,Cap_out]= Coestimation_4_cell (V_cell,I_cell,batt_param)

n_cells=4;
gamma = 0.98; 
Ts=0.1;
lambda=0.002;
alpha=0.98;

R0_matrix = batt_param.r0;         % Resistenza ohmica [Ohm]
R1_matrix = batt_param.r1;         % Resistenza RC [Ohm]
C1_matrix = batt_param.c1;          % Capacità RC [F]

SOC_grid =batt_param.soc(:);
OCV_tab  =batt_param.ocv(:);

        % Pre-calcola derivata OCV
        n_points = length(SOC_grid);
        dSOC = SOC_grid(2) - SOC_grid(1);
        dOCV_temp = diff(OCV_tab) / dSOC;
        dOCV_tab = zeros(n_points, 1);
        dOCV_tab(1) = dOCV_temp(1);
        for i = 2:n_points-1
            dOCV_tab(i) = dOCV_temp(i);
        end
        dOCV_tab(n_points) = dOCV_temp(n_points-1);


persistent init V_prec I_prec theta P_theta phi 
persistent x P Q R

if isempty(init)
    init=true;
    P_theta=zeros(4,4,n_cells);
    theta=zeros(4,n_cells);
    
    x= zeros(2,n_cells);
    P= zeros(2,2,n_cells);
    Q= zeros(2,2,n_cells);
    R= zeros(1,n_cells);


    for c=1:n_cells
        theta=eye(4)*1e3;
        V_prec=V_cell;
        I_prec=I_cell;
        
        SOC0=1;
        C0 = batt_param.c_cell(c);

        

        % ESTRAGGO LA RIGA k DALLA MATRICE E FACCIO L'INTERPOLAZIONE
        R0_row = R0_matrix(c, :);  % Riga k, vettore [1 x 21]
        R1_row = R1_matrix(c, :);  % Riga k, vettore [1 x 21]
        C1_row = C1_matrix(c, :);  % Riga k, vettore [1 x 21]
        
        % Converte a colonna per interp1
        R0_col = R0_row(:);  % [21 x 1]
        R1_col = R1_row(:);  % [21 x 1]
        C1_col = C1_row(:);  % [21 x 1]

        % Interpolazione
        R0_0 = interp1(SOC_grid, R0_col, SOC0, 'linear', 'extrap');
        Rp_0 = interp1(SOC_grid, R1_col, SOC0, 'linear', 'extrap');
        Cp_0 = interp1(SOC_grid, C1_col, SOC0, 'linear', 'extrap');
        OCV0 = interp1(SOC_grid, OCV_tab, SOC0, 'linear', 'extrap');

        alpha1 = exp(-Ts/(Rp_0*Cp_0));
        alpha3 = -R0_0;
        alpha4 = alpha1*R0_0 - (1-alpha1)*Rp_0;
        alpha2 = (1-alpha1)*OCV0;



        theta(:,c) = [alpha1; alpha2; alpha3; alpha4];
        P_theta(:,:,c) = eye(4)*1e3;
        
        x(:,c) = [SOC0;C0];
        P(:,:,c) = diag([1 1]);
        Q(:,:,c) = diag([1e-3 1e-3]);
        R(c)=1e1;

    end

end

SOC_out= zeros(n_cells,1);
Cap_out=zeros(n_cells,1);

for c=1:n_cells
    %% FFRLS
    y=V_cell;
    phi=[V_prec(c), 1, I_cell(c), I_prec(c)];
    
    Pth = P_theta(:,:,c);
    th = theta(:,c);
    
    %Time update

    K_theta = Pth*phi'/(phi*Pth*phi' + gamma);
    Pth=Pth*(eye(4) - K_theta*phi)/gamma;

    %Measurement update
    err = y - phi*th;
    th = th + K_theta.*err;

    theta(:,c) = th;
    P_theta(:,:,c) = Pth;
    
    Vocv=th(2)/(1-th(1));

    %% IAEKF
    
    SOCk=x(1,c);
    Ck= x(2,c);
    
    Pk=P(:,:,c);
    Qk=Q(:,:,c);
    Rk=R(c);

    SOC_prev=SOCk -(Ts*I_prec(c))/(3600*Ck);
    

    A = [1, (Ts*I_prec(c))/(3600*Ck^2);
        0,  1];
    OCV  = interp1(SOC_grid, OCV_tab, SOC_prev,"linear","extrap");
    dOCV= interp1(SOC_grid, dOCV_tab, SOC_prev, 'linear', 'extrap');
    
    C = [dOCV (dOCV*Ts*I_prec(c))/(3600*Ck^2)];
    
    P_prev = A * Pk * A' + Qk;

    K = Pk * C'/(C*Pk*C' + Rk);

    dk=Vocv - OCV;

    if dk>0.45
        x(:,c)=x(:,c) + K*dk;
    else
        x(:,c)=x(:,c) + lambda*K*dk;
    end
    
    Pk = (eye(2) - K*C)*P_prev;
    
    OCVmis=interp1(SOC_grid, OCV_tab, x(1,c),"linear","extrap");
    
    err=Vocv-OCVmis;

    Q(:,:,c)=Qk*alpha + (1-alpha)*(K*dk*dk'*K');

    R(c)= alpha*Rk + (1-alpha)*(err*err' + C* P_prev* C');

    P(:,:,c)=Pk;

    SOC_out(c)=x(1,c);
    Cap_out(c)=x(2,c);
end
V_prec=V_cell;
I_prec=I_cell;
end

== matlab function BMS_SOC/MATLAB Function5 ==
  settings: updateMethod=DISCRETE  sampleTime=0.1
  data: SOC_cells input; bal_cmd output; V_cells input; I_pack input; I_transfer output; batt_param parameter
function [bal_cmd, I_transfer] = BAL(SOC_cells, V_cells, I_pack, batt_param)

    n_cells = 4;
    
    I_bal_max = batt_param.I_bal_max;
    eta_dcdc = batt_param.eta_dcdc;
    SOC_threshold = batt_param.SOC_threshold;
    V_min_bal = batt_param.V_min_bal;
    V_max_bal = batt_param.V_max_bal;
    
    bal_cmd = zeros(4, 1);
    I_transfer = zeros(4, 1);
    
    % Trova SOC max e min
    SOC_min = SOC_cells(1);
    SOC_max = SOC_cells(1);
    idx_min = 1;
    idx_max = 1;
    
    for k = 1:n_cells
        if SOC_cells(k) < SOC_min
            SOC_min = SOC_cells(k);
            idx_min = k;
        end
        if SOC_cells(k) > SOC_max
            SOC_max = SOC_cells(k);
            idx_max = k;
        end
    end
    
    SOC_range = SOC_max - SOC_min;
    
    % Bilancia se necessario
    if SOC_range > SOC_threshold
        
        V_source = V_cells(idx_max);
        V_dest = V_cells(idx_min);
        
        safe = (V_source > V_min_bal) && (V_source < V_max_bal) && ... 
               (V_dest > V_min_bal) && (V_dest < V_max_bal);
        
        if safe
            I_bal = min(5 * SOC_range * I_bal_max, I_bal_max);
            
            bal_cmd(idx_max) = 1;
            I_transfer(idx_max) = I_bal;
            
            bal_cmd(idx_min) = -1;
            I_transfer(idx_min) = -I_bal * eta_dcdc;
        end
    end
    
end
